simulink model "PUMA_kinematics"  (R2016a)
settings: Solver=VariableStepAuto  StartTime=0.0  StopTime=10.0  RelTol=1e-3
values from neighbouring files (symbols this model uses):
  a2 = 320    [Puma_data.m]
  a3 = 0    [Puma_data.m]
  a4 = 0    [Puma_data.m]
  a5 = 0    [Puma_data.m]
  a6 = 0    [Puma_data.m]
  alpha2 = 0    [Puma_data.m]
  alpha3 = 90    [Puma_data.m]
  alpha4 = -90    [Puma_data.m]
  alpha5 = 90    [Puma_data.m]
  alpha6 = 0    [Puma_data.m]
  ceta2 = 0    [Puma_data.m]
  ceta3 = 0    [Puma_data.m]
  ceta4 = 0    [Puma_data.m]
  ceta5 = 0    [Puma_data.m]
  ceta6 = 0    [Puma_data.m]
  d2 = -55    [Puma_data.m]
  d3 = 0    [Puma_data.m]
  d4 = 350    [Puma_data.m]
  d5 = 0    [Puma_data.m]
  d6 = 140    [Puma_data.m]
undefined symbols (not defined in the file or in its folder): a1, alpha1, ceta1, d1
settings Model: Creator=Amr  LastModifiedBy=Amr

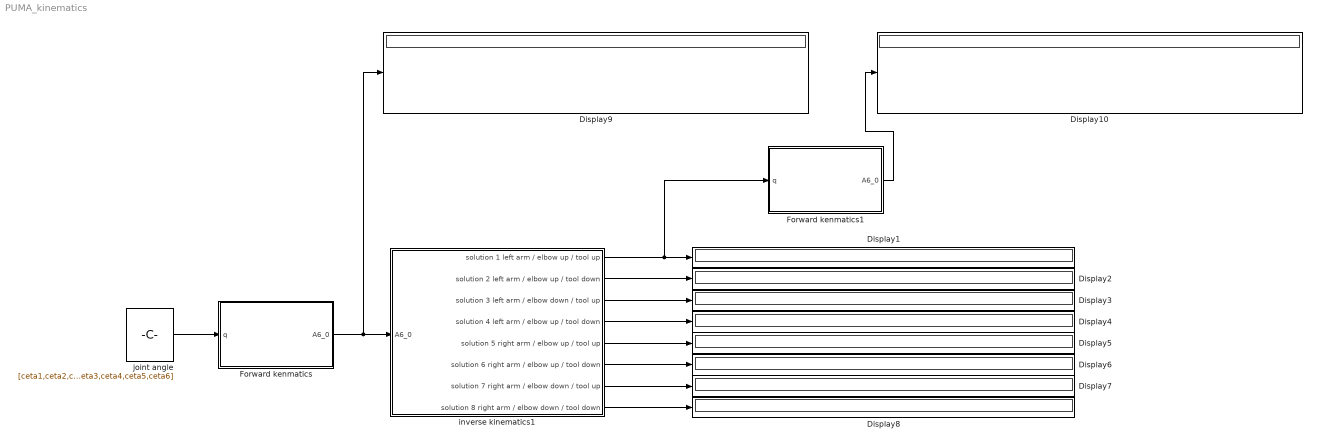
== system PUMA_kinematics ==
  Display{1..10} (10 alike) : Display
  Forward kenmatics : Subsystem
  Forward kenmatics1 : Subsystem
  inverse kinematics1 : Subsystem
  joint angle : Constant  Value=[ceta1,ceta2,ceta3,ceta4,ceta5,ceta6]
  wires:
  joint angle/1 -> Forward kenmatics/1(q)
  inverse kinematics1/1(solution 1 left arm / elbow up / tool up) -> Forward kenmatics1/1(q), Display1/1
  inverse kinematics1/4(solution 4 left arm / elbow up / tool down) -> Display4/1
  inverse kinematics1/3(solution 3 left arm / elbow down / tool up) -> Display3/1
  inverse kinematics1/2(solution 2 left arm / elbow up / tool down) -> Display2/1
  inverse kinematics1/6(solution 6 right arm / elbow up / tool down) -> Display6/1
  inverse kinematics1/7(solution 7 right arm / elbow down / tool up) -> Display7/1
  Forward kenmatics/1(A6_0) -> Display9/1, inverse kinematics1/1(A6_0)
  inverse kinematics1/8(solution 8 right arm / elbow down / tool down) -> Display8/1
  Forward kenmatics1/1(A6_0) -> Display10/1
  inverse kinematics1/5(solution 5 right arm / elbow up / tool up) -> Display5/1

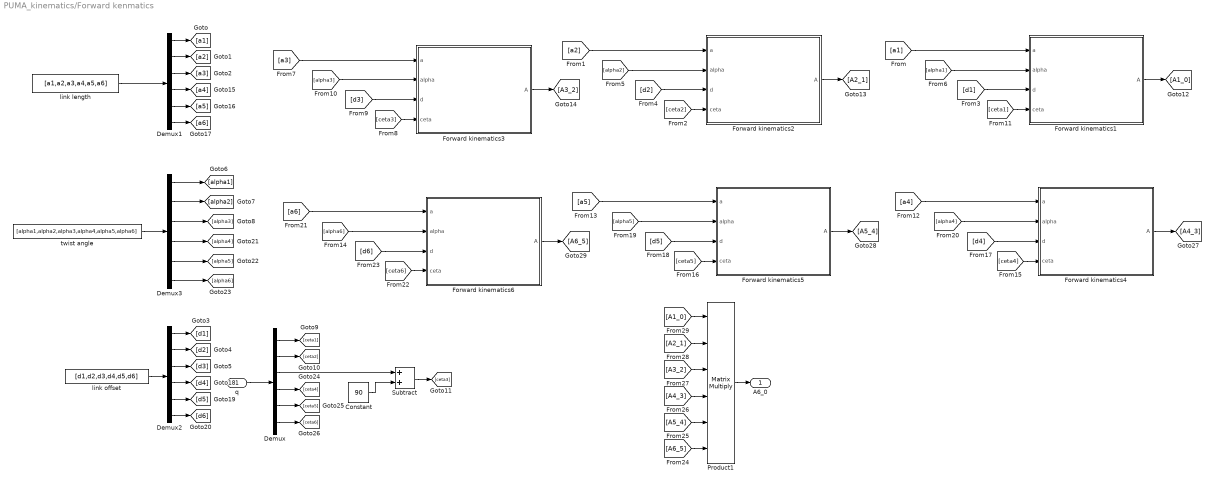
== system PUMA_kinematics/Forward kenmatics ==
  q : Inport
  " Forward kinematics1" : MATLAB Function  TreatAsAtomicUnit=on
  " Forward kinematics2" : MATLAB Function  TreatAsAtomicUnit=on
  " Forward kinematics3" : MATLAB Function  TreatAsAtomicUnit=on
  " Forward kinematics4" : MATLAB Function  TreatAsAtomicUnit=on
  " Forward kinematics5" : MATLAB Function  TreatAsAtomicUnit=on
  " Forward kinematics6" : MATLAB Function  TreatAsAtomicUnit=on
  Constant : Constant  Value=90
  Demux{,1..3} (4 alike) : Demux  Outputs=6
  Product1 : Product  Inputs=6  Multiplication=Matrix(*)
  Subtract : Sum
  link length : Constant  Value=[a1,a2,a3,a4,a5,a6]
  link offset : Constant  Value=[d1,d2,d3,d4,d5,d6]
  twist angle : Constant  Value=[alpha1,alpha2,alpha3,alpha4,alpha5,alpha6]
  A6_0 : Outport
  wires:
  Demux2/4 -> [d4]
  " Forward kinematics3"/1(A) -> [A3_2]
  Demux2/6 -> [d6]
  Demux1/6 -> [a6]
  Demux1/4 -> [a4]
  Demux/4 -> [ceta4]
  Demux/5 -> [ceta5]
  Demux1/5 -> [a5]
  " Forward kinematics1"/1(A) -> [A1_0]
  [d2] -> " Forward kinematics2"/3(d)
  [a2] -> " Forward kinematics2"/1(a)
  [alpha2] -> " Forward kinematics2"/2(alpha)
  [ceta2] -> " Forward kinematics2"/4(ceta)
  [ceta4] -> " Forward kinematics4"/4(ceta)
  [a5] -> " Forward kinematics5"/1(a)
  [a6] -> " Forward kinematics6"/1(a)
  [d6] -> " Forward kinematics6"/3(d)
  [alpha4] -> " Forward kinematics4"/2(alpha)
  [a4] -> " Forward kinematics4"/1(a)
  [alpha5] -> " Forward kinematics5"/2(alpha)
  [ceta5] -> " Forward kinematics5"/4(ceta)
  [d4] -> " Forward kinematics4"/3(d)
  [d5] -> " Forward kinematics5"/3(d)
  [alpha6] -> " Forward kinematics6"/2(alpha)
  " Forward kinematics6"/1(A) -> [A6_5]
  " Forward kinematics5"/1(A) -> [A5_4]
  " Forward kinematics4"/1(A) -> [A4_3]
  [ceta6] -> " Forward kinematics6"/4(ceta)
  Demux3/6 -> [alpha6]
  Demux2/5 -> [d5]
  " Forward kinematics2"/1(A) -> [A2_1]
  Demux3/5 -> [alpha5]
  Demux3/4 -> [alpha4]
  Demux/6 -> [ceta6]
  [d3] -> " Forward kinematics3"/3(d)
  [ceta3] -> " Forward kinematics3"/4(ceta)
  [a3] -> " Forward kinematics3"/1(a)
  [alpha3] -> " Forward kinematics3"/2(alpha)
  Demux1/1 -> [a1]
  Demux1/2 -> [a2]
  q/1 -> Demux/1
  Demux1/3 -> [a3]
  link offset/1 -> Demux2/1
  Demux2/1 -> [d1]
  Product1/1 -> A6_0/1
  Demux/1 -> [ceta1]
  [ceta1] -> " Forward kinematics1"/4(ceta)
  twist angle/1 -> Demux3/1
  Demux3/1 -> [alpha1]
  Demux2/3 -> [d3]
  [a1] -> " Forward kinematics1"/1(a)
  Demux/2 -> [ceta2]
  Demux2/2 -> [d2]
  [d1] -> " Forward kinematics1"/3(d)
  link length/1 -> Demux1/1
  Demux3/2 -> [alpha2]
  [alpha1] -> " Forward kinematics1"/2(alpha)
  Demux3/3 -> [alpha3]
  [A5_4] -> Product1/5
  [A6_5] -> Product1/6
  [A1_0] -> Product1/1
  [A2_1] -> Product1/2
  [A4_3] -> Product1/4
  Constant/1 -> Subtract/2
  Subtract/1 -> [ceta3]
  Demux/3 -> Subtract/1
  [A3_2] -> Product1/3

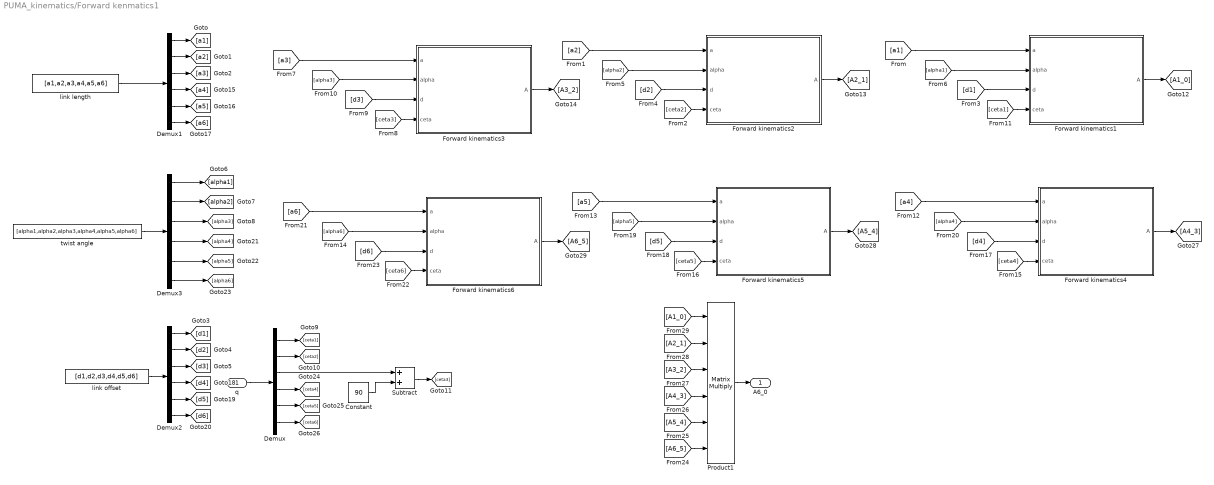
== system PUMA_kinematics/Forward kenmatics1 ==
  q : Inport
  " Forward kinematics1" : MATLAB Function  TreatAsAtomicUnit=on
  " Forward kinematics2" : MATLAB Function  TreatAsAtomicUnit=on
  " Forward kinematics3" : MATLAB Function  TreatAsAtomicUnit=on
  " Forward kinematics4" : MATLAB Function  TreatAsAtomicUnit=on
  " Forward kinematics5" : MATLAB Function  TreatAsAtomicUnit=on
  " Forward kinematics6" : MATLAB Function  TreatAsAtomicUnit=on
  Constant : Constant  Value=90
  Demux{,1..3} (4 alike) : Demux  Outputs=6
  Product1 : Product  Inputs=6  Multiplication=Matrix(*)
  Subtract : Sum
  link length : Constant  Value=[a1,a2,a3,a4,a5,a6]
  link offset : Constant  Value=[d1,d2,d3,d4,d5,d6]
  twist angle : Constant  Value=[alpha1,alpha2,alpha3,alpha4,alpha5,alpha6]
  A6_0 : Outport
  wires:
  Demux2/4 -> [d4]
  " Forward kinematics3"/1(A) -> [A3_2]
  Demux2/6 -> [d6]
  Demux1/6 -> [a6]
  Demux1/4 -> [a4]
  Demux/4 -> [ceta4]
  Demux/5 -> [ceta5]
  Demux1/5 -> [a5]
  " Forward kinematics1"/1(A) -> [A1_0]
  [d2] -> " Forward kinematics2"/3(d)
  [a2] -> " Forward kinematics2"/1(a)
  [alpha2] -> " Forward kinematics2"/2(alpha)
  [ceta2] -> " Forward kinematics2"/4(ceta)
  [ceta4] -> " Forward kinematics4"/4(ceta)
  [a5] -> " Forward kinematics5"/1(a)
  [a6] -> " Forward kinematics6"/1(a)
  [d6] -> " Forward kinematics6"/3(d)
  [alpha4] -> " Forward kinematics4"/2(alpha)
  [a4] -> " Forward kinematics4"/1(a)
  [alpha5] -> " Forward kinematics5"/2(alpha)
  [ceta5] -> " Forward kinematics5"/4(ceta)
  [d4] -> " Forward kinematics4"/3(d)
  [d5] -> " Forward kinematics5"/3(d)
  [alpha6] -> " Forward kinematics6"/2(alpha)
  " Forward kinematics6"/1(A) -> [A6_5]
  " Forward kinematics5"/1(A) -> [A5_4]
  " Forward kinematics4"/1(A) -> [A4_3]
  [ceta6] -> " Forward kinematics6"/4(ceta)
  Demux3/6 -> [alpha6]
  Demux2/5 -> [d5]
  " Forward kinematics2"/1(A) -> [A2_1]
  Demux3/5 -> [alpha5]
  Demux3/4 -> [alpha4]
  Demux/6 -> [ceta6]
  [d3] -> " Forward kinematics3"/3(d)
  [ceta3] -> " Forward kinematics3"/4(ceta)
  [a3] -> " Forward kinematics3"/1(a)
  [alpha3] -> " Forward kinematics3"/2(alpha)
  Demux1/1 -> [a1]
  Demux1/2 -> [a2]
  q/1 -> Demux/1
  Demux1/3 -> [a3]
  link offset/1 -> Demux2/1
  Demux2/1 -> [d1]
  Product1/1 -> A6_0/1
  Demux/1 -> [ceta1]
  [ceta1] -> " Forward kinematics1"/4(ceta)
  twist angle/1 -> Demux3/1
  Demux3/1 -> [alpha1]
  Demux2/3 -> [d3]
  [a1] -> " Forward kinematics1"/1(a)
  Demux/2 -> [ceta2]
  Demux2/2 -> [d2]
  [d1] -> " Forward kinematics1"/3(d)
  link length/1 -> Demux1/1
  Demux3/2 -> [alpha2]
  [alpha1] -> " Forward kinematics1"/2(alpha)
  Demux3/3 -> [alpha3]
  [A5_4] -> Product1/5
  [A6_5] -> Product1/6
  [A1_0] -> Product1/1
  [A2_1] -> Product1/2
  [A4_3] -> Product1/4
  Constant/1 -> Subtract/2
  Subtract/1 -> [ceta3]
  Demux/3 -> Subtract/1
  [A3_2] -> Product1/3

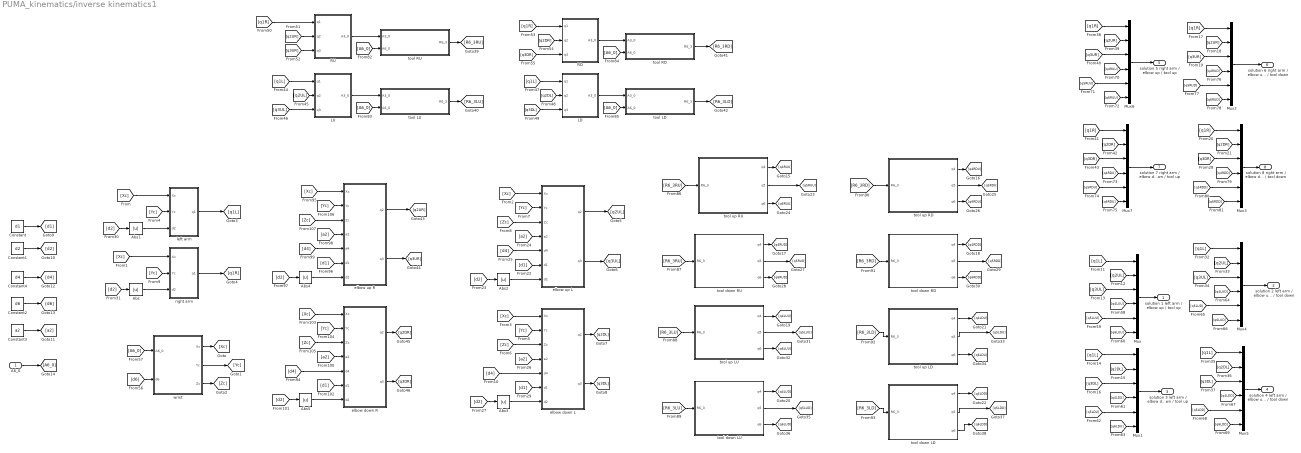
== system PUMA_kinematics/inverse kinematics1 ==
  A6_0 : Inport
  Abs{,1..5} (6 alike) : Abs
  Constant : Constant  Value=d1
  Constant1 : Constant  Value=d2
  Constant2 : Constant  Value=d6
  Constant3 : Constant  Value=a2
  Constant4 : Constant  Value=d4
  LD : Subsystem
  LU : Subsystem
  Mux{,1..7} (8 alike) : Mux  Inputs=6
  RD : Subsystem
  RU : Subsystem
  elbow down L : MATLAB Function  TreatAsAtomicUnit=on
  elbow down R : MATLAB Function  TreatAsAtomicUnit=on
  elbow up L : MATLAB Function  TreatAsAtomicUnit=on
  elbow up R : MATLAB Function  TreatAsAtomicUnit=on
  left arm : MATLAB Function  TreatAsAtomicUnit=on
  right arm : MATLAB Function  TreatAsAtomicUnit=on
  tool LD : MATLAB Function  TreatAsAtomicUnit=on
  tool LU : MATLAB Function  TreatAsAtomicUnit=on
  tool RD : MATLAB Function  TreatAsAtomicUnit=on
  tool RU : MATLAB Function  TreatAsAtomicUnit=on
  tool down LD : MATLAB Function  TreatAsAtomicUnit=on
  tool down LU : MATLAB Function  TreatAsAtomicUnit=on
  tool down RD : MATLAB Function  TreatAsAtomicUnit=on
  tool down RU : MATLAB Function  TreatAsAtomicUnit=on
  tool up LD : MATLAB Function  TreatAsAtomicUnit=on
  tool up LU : MATLAB Function  TreatAsAtomicUnit=on
  tool up RD : MATLAB Function  TreatAsAtomicUnit=on
  tool up RU : MATLAB Function  TreatAsAtomicUnit=on
  wrist : MATLAB Function  TreatAsAtomicUnit=on
  solution 1 left arm / elbow up / tool up : Outport
  solution 2 left arm / elbow up / tool down : Outport  Port=2
  solution 3 left arm / elbow down / tool up : Outport  Port=3
  solution 4 left arm / elbow up / tool down : Outport  Port=4
  solution 5 right arm / elbow up / tool up : Outport  Port=5
  solution 6 right arm / elbow up / tool down : Outport  Port=6
  solution 7 right arm / elbow down / tool up : Outport  Port=7
  solution 8 right arm / elbow down / tool down : Outport  Port=8
  wires:
  [Yc] -> right arm/2(Yc)
  left arm/1(q1) -> [q1L]
  [Yc] -> left arm/2(Yc)
  [d6] -> wrist/2(d6)
  wrist/2(Yc) -> [Yc]
  Constant/1 -> [d1]
  Constant3/1 -> [a2]
  [A6_0] -> wrist/1(A6_0)
  A6_0/1 -> [A6_0]
  Constant4/1 -> [d4]
  Constant1/1 -> [d2]
  Constant2/1 -> [d6]
  right arm/1(q1) -> [q1R]
  wrist/3(Zc) -> [Zc]
  [Xc] -> right arm/1(Xc)
  [Xc] -> left arm/1(Xc)
  wrist/1(Xc) -> [Xc]
  [d2] -> Abs/1
  Abs/1 -> right arm/3(d2)
  [d2] -> Abs1/1
  Abs1/1 -> left arm/3(d2)
  [d4] -> elbow up L/5(d4)
  [Xc] -> elbow up L/1(Xc)
  [d1] -> elbow up L/6(d1)
  [a2] -> elbow up L/4(a2)
  [Zc] -> elbow up L/3(Zc)
  [Yc] -> elbow up L/2(Yc)
  [d2] -> Abs2/1
  Abs2/1 -> elbow up L/7(d2)
  elbow up L/2(q3) -> [q3UL]
  elbow up L/1(q2) -> [q2UL]
  elbow down L/2(q3) -> [q3DL]
  elbow down L/1(q2) -> [q2DL]
  [a2] -> elbow down L/4(a2)
  [d4] -> elbow down L/5(d4)
  [Xc] -> elbow down L/1(Xc)
  [Yc] -> elbow down L/2(Yc)
  [d1] -> elbow down L/6(d1)
  [Zc] -> elbow down L/3(Zc)
  Abs3/1 -> elbow down L/7(d2)
  [d2] -> Abs3/1
  [q3UL] -> LU/3(q3)
  [q1R] -> RD/1(q1)
  [q3DR] -> RD/3(q3)
  [q2DR] -> RD/2(q2)
  [q2UL] -> LU/2(q2)
  RU/1(A3_0) -> tool RU/1(A3_0)
  LU/1(A3_0) -> tool LU/1(A3_0)
  RD/1(A3_0) -> tool RD/1(A3_0)
  LD/1(A3_0) -> tool LD/1(A3_0)
  [A6_0] -> tool RU/2(A6_0)
  [A6_0] -> tool LU/2(A6_0)
  [A6_0] -> tool RD/2(A6_0)
  [A6_0] -> tool LD/2(A6_0)
  tool RU/1(R6_3) -> [R6_3RU]
  tool LU/1(R6_3) -> [R6_3LU]
  [q1L] -> LU/1(q1)
  [q1R] -> RU/1(q1)
  [q2UR] -> RU/2(q2)
  [q3UR] -> RU/3(q3)
  [q3DL] -> LD/3(q3)
  [q1L] -> LD/1(q1)
  [q2DL] -> LD/2(q2)
  tool RD/1(R6_3) -> [R6_3RD]
  tool up RU/1(q4) -> [q4RUU]
  tool up RU/2(q5) -> [q5RUU]
  tool up RU/3(q6) -> [q6RUU]
  tool LD/1(R6_3) -> [R6_3LD]
  [R6_3RU] -> tool up RU/1(R6_3)
  tool up LD/2(q5) -> [q5LDU]
  tool up LD/1(q4) -> [q4LDU]
  tool down LD/2(q5) -> [q5LDD]
  tool up LD/3(q6) -> [q6LDU]
  tool down RD/1(q4) -> [q4RDD]
  tool down RD/2(q5) -> [q5RDD]
  tool down RD/3(q6) -> [q6RDD]
  tool up RD/1(q4) -> [q4RDU]
  tool up RD/3(q6) -> [q6RDU]
  tool up RD/2(q5) -> [q5RDU]
  [R6_3RD] -> tool down RD/1(R6_3)
  [R6_3RD] -> tool up RD/1(R6_3)
  [R6_3LD] -> tool up LD/1(R6_3)
  [R6_3LD] -> tool down LD/1(R6_3)
  tool down LU/1(q4) -> [q4LUD]
  tool down LU/2(q5) -> [q5LUD]
  tool down LU/3(q6) -> [q6LUD]
  tool down RU/1(q4) -> [q4RUD]
  tool up LU/1(q4) -> [q4LUU]
  tool down RU/3(q6) -> [q6RUD]
  tool down RU/2(q5) -> [q5RUD]
  tool up LU/2(q5) -> [q5LUU]
  tool up LU/3(q6) -> [q6LUU]
  [R6_3RU] -> tool down RU/1(R6_3)
  [R6_3LU] -> tool up LU/1(R6_3)
  [R6_3LU] -> tool down LU/1(R6_3)
  [q3DL] -> Mux1/3
  [q3UR] -> Mux2/3
  [q2UR] -> Mux2/2
  [q1R] -> Mux2/1
  [q4LDD] -> Mux5/4
  [q5LDD] -> Mux5/5
  [q6LDD] -> Mux5/6
  [q4LUD] -> Mux4/4
  [q5LUU] -> Mux/5
  [q4LUU] -> Mux/4
  [q6LUU] -> Mux/6
  [q5LUD] -> Mux4/5
  [q5RUU] -> Mux6/5
  [q6LUD] -> Mux4/6
  [q4RUU] -> Mux6/4
  [q6RUU] -> Mux6/6
  [q4RUD] -> Mux2/4
  [q6RUD] -> Mux2/6
  [q5RUD] -> Mux2/5
  [q1R] -> Mux3/1
  [q2DL] -> Mux1/2
  [q3UL] -> Mux/3
  [q5LDU] -> Mux1/5
  [q6LDU] -> Mux1/6
  [q4LDU] -> Mux1/4
  [q3DR] -> Mux3/3
  Mux/1 -> solution 1 left arm / elbow up / tool up/1
  [q1L] -> Mux1/1
  [q3DR] -> Mux7/3
  [q2DL] -> Mux5/2
  [q1R] -> Mux7/1
  [q3UR] -> Mux6/3
  [q1R] -> Mux6/1
  [q1L] -> Mux5/1
  [q2DR] -> Mux7/2
  [q3UL] -> Mux4/3
  [q2UR] -> Mux6/2
  [q3DL] -> Mux5/3
  [q1L] -> Mux4/1
  [q2UL] -> Mux4/2
  [q2DR] -> Mux3/2
  [q1L] -> Mux/1
  [q2UL] -> Mux/2
  Mux4/1 -> solution 2 left arm / elbow up / tool down/1
  Mux1/1 -> solution 3 left arm / elbow down / tool up/1
  Mux5/1 -> solution 4 left arm / elbow up / tool down/1
  Mux6/1 -> solution 5 right arm / elbow up / tool up/1
  Mux2/1 -> solution 6 right arm / elbow up / tool down/1
  Mux7/1 -> solution 7 right arm / elbow down / tool up/1
  Mux3/1 -> solution 8 right arm / elbow down / tool down/1
  [q4RDU] -> Mux7/4
  [q5RDU] -> Mux7/5
  [q6RDU] -> Mux7/6
  [q6RDD] -> Mux3/6
  [q5RDD] -> Mux3/5
  [q4RDD] -> Mux3/4
  tool down LD/1(q4) -> [q4LDD]
  tool down LD/3(q6) -> [q6LDD]
  [d4] -> elbow up R/5(d4)
  [Xc] -> elbow up R/1(Xc)
  [d1] -> elbow up R/6(d1)
  [a2] -> elbow up R/4(a2)
  [Zc] -> elbow up R/3(Zc)
  [Yc] -> elbow up R/2(Yc)
  [d2] -> Abs4/1
  Abs4/1 -> elbow up R/7(d2)
  elbow up R/2(q3) -> [q3UR]
  elbow up R/1(q2) -> [q2UR]
  elbow down R/2(q3) -> [q3DR]
  elbow down R/1(q2) -> [q2DR]
  [a2] -> elbow down R/4(a2)
  [d4] -> elbow down R/5(d4)
  [Xc] -> elbow down R/1(Xc)
  [Yc] -> elbow down R/2(Yc)
  [d1] -> elbow down R/6(d1)
  [Zc] -> elbow down R/3(Zc)
  Abs5/1 -> elbow down R/7(d2)
  [d2] -> Abs5/1

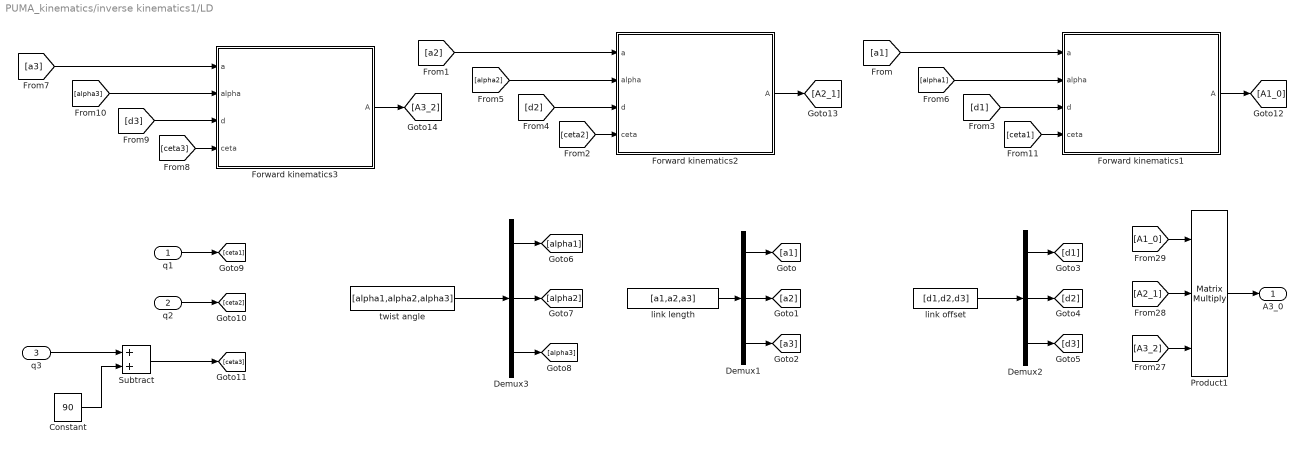
== system PUMA_kinematics/inverse kinematics1/LD ==
  q1 : Inport
  q2 : Inport  Port=2
  q3 : Inport  Port=3
  " Forward kinematics1" : MATLAB Function  TreatAsAtomicUnit=on
  " Forward kinematics2" : MATLAB Function  TreatAsAtomicUnit=on
  " Forward kinematics3" : MATLAB Function  TreatAsAtomicUnit=on
  Constant : Constant  Value=90
  Demux1 : Demux  Outputs=3
  Demux2 : Demux  Outputs=3
  Demux3 : Demux  Outputs=3
  Product1 : Product  Inputs=3  Multiplication=Matrix(*)
  Subtract : Sum
  link length : Constant  Value=[a1,a2,a3]
  link offset : Constant  Value=[d1,d2,d3]
  twist angle : Constant  Value=[alpha1,alpha2,alpha3]
  A3_0 : Outport
  wires:
  " Forward kinematics3"/1(A) -> [A3_2]
  " Forward kinematics1"/1(A) -> [A1_0]
  [d2] -> " Forward kinematics2"/3(d)
  [a2] -> " Forward kinematics2"/1(a)
  [alpha2] -> " Forward kinematics2"/2(alpha)
  [ceta2] -> " Forward kinematics2"/4(ceta)
  " Forward kinematics2"/1(A) -> [A2_1]
  [d3] -> " Forward kinematics3"/3(d)
  [ceta3] -> " Forward kinematics3"/4(ceta)
  [a3] -> " Forward kinematics3"/1(a)
  [alpha3] -> " Forward kinematics3"/2(alpha)
  Demux1/1 -> [a1]
  Demux1/2 -> [a2]
  Demux1/3 -> [a3]
  link offset/1 -> Demux2/1
  Demux2/1 -> [d1]
  Product1/1 -> A3_0/1
  [ceta1] -> " Forward kinematics1"/4(ceta)
  twist angle/1 -> Demux3/1
  Demux3/1 -> [alpha1]
  Demux2/3 -> [d3]
  [a1] -> " Forward kinematics1"/1(a)
  Demux2/2 -> [d2]
  [d1] -> " Forward kinematics1"/3(d)
  link length/1 -> Demux1/1
  Demux3/2 -> [alpha2]
  [alpha1] -> " Forward kinematics1"/2(alpha)
  Demux3/3 -> [alpha3]
  [A3_2] -> Product1/3
  [A1_0] -> Product1/1
  [A2_1] -> Product1/2
  q1/1 -> [ceta1]
  q2/1 -> [ceta2]
  Constant/1 -> Subtract/2
  Subtract/1 -> [ceta3]
  q3/1 -> Subtract/1

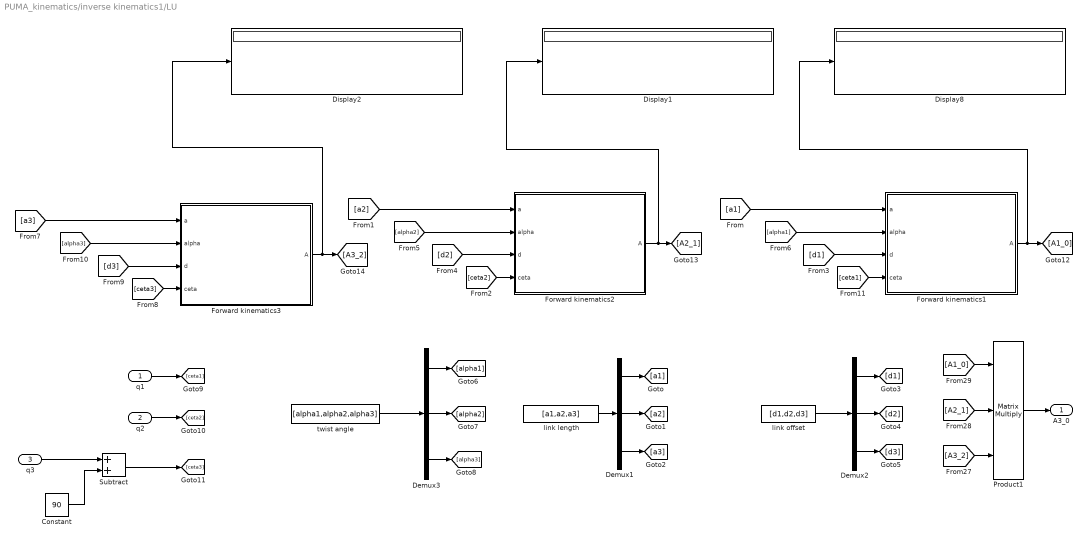
== system PUMA_kinematics/inverse kinematics1/LU ==
  q1 : Inport
  q2 : Inport  Port=2
  q3 : Inport  Port=3
  " Forward kinematics1" : MATLAB Function  TreatAsAtomicUnit=on
  " Forward kinematics2" : MATLAB Function  TreatAsAtomicUnit=on
  " Forward kinematics3" : MATLAB Function  TreatAsAtomicUnit=on
  Constant : Constant  Value=90
  Demux1 : Demux  Outputs=3
  Demux2 : Demux  Outputs=3
  Demux3 : Demux  Outputs=3
  Display1 : Display
  Display2 : Display
  Display8 : Display
  Product1 : Product  Inputs=3  Multiplication=Matrix(*)
  Subtract : Sum
  link length : Constant  Value=[a1,a2,a3]
  link offset : Constant  Value=[d1,d2,d3]
  twist angle : Constant  Value=[alpha1,alpha2,alpha3]
  A3_0 : Outport
  wires:
  " Forward kinematics3"/1(A) -> Display2/1, [A3_2]
  " Forward kinematics1"/1(A) -> Display8/1, [A1_0]
  [d2] -> " Forward kinematics2"/3(d)
  [a2] -> " Forward kinematics2"/1(a)
  [alpha2] -> " Forward kinematics2"/2(alpha)
  [ceta2] -> " Forward kinematics2"/4(ceta)
  [d3] -> " Forward kinematics3"/3(d)
  [ceta3] -> " Forward kinematics3"/4(ceta)
  [a3] -> " Forward kinematics3"/1(a)
  [alpha3] -> " Forward kinematics3"/2(alpha)
  Demux1/1 -> [a1]
  Demux1/2 -> [a2]
  Demux1/3 -> [a3]
  link offset/1 -> Demux2/1
  Demux2/1 -> [d1]
  Product1/1 -> A3_0/1
  [ceta1] -> " Forward kinematics1"/4(ceta)
  twist angle/1 -> Demux3/1
  Demux3/1 -> [alpha1]
  Demux2/3 -> [d3]
  [a1] -> " Forward kinematics1"/1(a)
  Demux2/2 -> [d2]
  [d1] -> " Forward kinematics1"/3(d)
  link length/1 -> Demux1/1
  Demux3/2 -> [alpha2]
  [alpha1] -> " Forward kinematics1"/2(alpha)
  Demux3/3 -> [alpha3]
  [A3_2] -> Product1/3
  [A1_0] -> Product1/1
  [A2_1] -> Product1/2
  q1/1 -> [ceta1]
  q2/1 -> [ceta2]
  Constant/1 -> Subtract/2
  Subtract/1 -> [ceta3]
  q3/1 -> Subtract/1
  " Forward kinematics2"/1(A) -> [A2_1], Display1/1

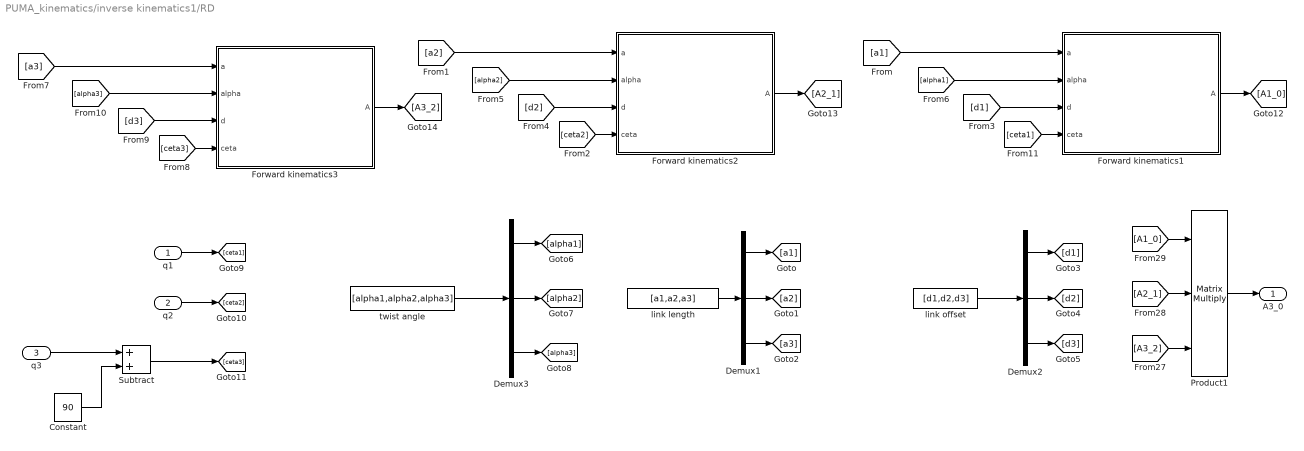
== system PUMA_kinematics/inverse kinematics1/RD ==
  q1 : Inport
  q2 : Inport  Port=2
  q3 : Inport  Port=3
  " Forward kinematics1" : MATLAB Function  TreatAsAtomicUnit=on
  " Forward kinematics2" : MATLAB Function  TreatAsAtomicUnit=on
  " Forward kinematics3" : MATLAB Function  TreatAsAtomicUnit=on
  Constant : Constant  Value=90
  Demux1 : Demux  Outputs=3
  Demux2 : Demux  Outputs=3
  Demux3 : Demux  Outputs=3
  Product1 : Product  Inputs=3  Multiplication=Matrix(*)
  Subtract : Sum
  link length : Constant  Value=[a1,a2,a3]
  link offset : Constant  Value=[d1,d2,d3]
  twist angle : Constant  Value=[alpha1,alpha2,alpha3]
  A3_0 : Outport
  wires:
  " Forward kinematics3"/1(A) -> [A3_2]
  " Forward kinematics1"/1(A) -> [A1_0]
  [d2] -> " Forward kinematics2"/3(d)
  [a2] -> " Forward kinematics2"/1(a)
  [alpha2] -> " Forward kinematics2"/2(alpha)
  [ceta2] -> " Forward kinematics2"/4(ceta)
  " Forward kinematics2"/1(A) -> [A2_1]
  [d3] -> " Forward kinematics3"/3(d)
  [ceta3] -> " Forward kinematics3"/4(ceta)
  [a3] -> " Forward kinematics3"/1(a)
  [alpha3] -> " Forward kinematics3"/2(alpha)
  Demux1/1 -> [a1]
  Demux1/2 -> [a2]
  Demux1/3 -> [a3]
  link offset/1 -> Demux2/1
  Demux2/1 -> [d1]
  Product1/1 -> A3_0/1
  [ceta1] -> " Forward kinematics1"/4(ceta)
  twist angle/1 -> Demux3/1
  Demux3/1 -> [alpha1]
  Demux2/3 -> [d3]
  [a1] -> " Forward kinematics1"/1(a)
  Demux2/2 -> [d2]
  [d1] -> " Forward kinematics1"/3(d)
  link length/1 -> Demux1/1
  Demux3/2 -> [alpha2]
  [alpha1] -> " Forward kinematics1"/2(alpha)
  Demux3/3 -> [alpha3]
  [A3_2] -> Product1/3
  [A1_0] -> Product1/1
  [A2_1] -> Product1/2
  q1/1 -> [ceta1]
  q2/1 -> [ceta2]
  Constant/1 -> Subtract/2
  Subtract/1 -> [ceta3]
  q3/1 -> Subtract/1

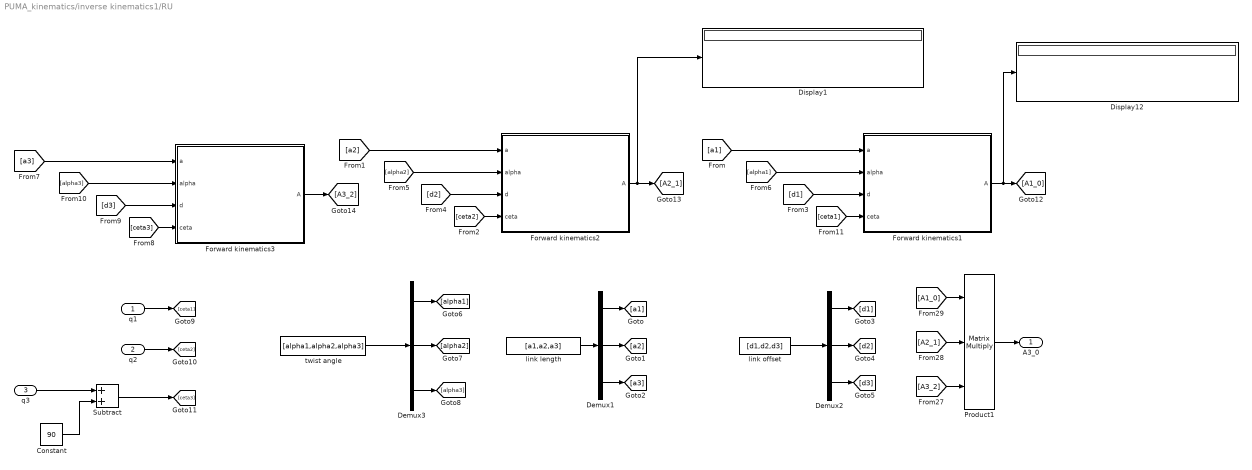
== system PUMA_kinematics/inverse kinematics1/RU ==
  q1 : Inport
  q2 : Inport  Port=2
  q3 : Inport  Port=3
  " Forward kinematics1" : MATLAB Function  TreatAsAtomicUnit=on
  " Forward kinematics2" : MATLAB Function  TreatAsAtomicUnit=on
  " Forward kinematics3" : MATLAB Function  TreatAsAtomicUnit=on
  Constant : Constant  Value=90
  Demux1 : Demux  Outputs=3
  Demux2 : Demux  Outputs=3
  Demux3 : Demux  Outputs=3
  Display1 : Display
  Display12 : Display
  Product1 : Product  Inputs=3  Multiplication=Matrix(*)
  Subtract : Sum
  link length : Constant  Value=[a1,a2,a3]
  link offset : Constant  Value=[d1,d2,d3]
  twist angle : Constant  Value=[alpha1,alpha2,alpha3]
  A3_0 : Outport
  wires:
  " Forward kinematics3"/1(A) -> [A3_2]
  " Forward kinematics1"/1(A) -> Display12/1, [A1_0]
  [d2] -> " Forward kinematics2"/3(d)
  [a2] -> " Forward kinematics2"/1(a)
  [alpha2] -> " Forward kinematics2"/2(alpha)
  [ceta2] -> " Forward kinematics2"/4(ceta)
  " Forward kinematics2"/1(A) -> Display1/1, [A2_1]
  [d3] -> " Forward kinematics3"/3(d)
  [ceta3] -> " Forward kinematics3"/4(ceta)
  [a3] -> " Forward kinematics3"/1(a)
  [alpha3] -> " Forward kinematics3"/2(alpha)
  Demux1/1 -> [a1]
  Demux1/2 -> [a2]
  Demux1/3 -> [a3]
  link offset/1 -> Demux2/1
  Demux2/1 -> [d1]
  Product1/1 -> A3_0/1
  [ceta1] -> " Forward kinematics1"/4(ceta)
  twist angle/1 -> Demux3/1
  Demux3/1 -> [alpha1]
  Demux2/3 -> [d3]
  [a1] -> " Forward kinematics1"/1(a)
  Demux2/2 -> [d2]
  [d1] -> " Forward kinematics1"/3(d)
  link length/1 -> Demux1/1
  Demux3/2 -> [alpha2]
  [alpha1] -> " Forward kinematics1"/2(alpha)
  Demux3/3 -> [alpha3]
  [A3_2] -> Product1/3
  [A1_0] -> Product1/1
  [A2_1] -> Product1/2
  q1/1 -> [ceta1]
  q2/1 -> [ceta2]
  Constant/1 -> Subtract/2
  Subtract/1 -> [ceta3]
  q3/1 -> Subtract/1

== matlab function PUMA_kinematics/Forward kenmatics/ Forward kinematics2 ==
  data: a input; alpha input; A output; d input; ceta input

function  A=fk_transformation_matrix(a,alpha,d,ceta )


A=[cosd(ceta) , (-1*sind(ceta)*cosd(alpha)) , (sind(ceta)*sind(alpha)) , (a*cosd(ceta)) ;...........................
    sind(ceta) , (cosd(ceta)*cosd(alpha)) ,(-1*cosd(ceta)*sind(alpha)) , (a*sind(ceta)) ;............................
    0 , sind(alpha) , cosd(alpha) , d ;..................................................................................
    0,0,0,1];

== matlab function PUMA_kinematics/Forward kenmatics/ Forward kinematics3 ==
  data: a input; alpha input; A output; d input; ceta input

function  A=fk_transformation_matrix(a,alpha,d,ceta )


A=[cosd(ceta) , (-1*sind(ceta)*cosd(alpha)) , (sind(ceta)*sind(alpha)) , (a*cosd(ceta)) ;...........................
    sind(ceta) , (cosd(ceta)*cosd(alpha)) ,(-1*cosd(ceta)*sind(alpha)) , (a*sind(ceta)) ;............................
    0 , sind(alpha) , cosd(alpha) , d ;..................................................................................
    0,0,0,1];

== matlab function PUMA_kinematics/Forward kenmatics/ Forward kinematics4 ==
  data: a input; alpha input; A output; d input; ceta input

function  A=fk_transformation_matrix(a,alpha,d,ceta )


A=[cosd(ceta) , (-1*sind(ceta)*cosd(alpha)) , (sind(ceta)*sind(alpha)) , (a*cosd(ceta)) ;...........................
    sind(ceta) , (cosd(ceta)*cosd(alpha)) ,(-1*cosd(ceta)*sind(alpha)) , (a*sind(ceta)) ;............................
    0 , sind(alpha) , cosd(alpha) , d ;..................................................................................
    0,0,0,1];

== matlab function PUMA_kinematics/Forward kenmatics/ Forward kinematics5 ==
  data: a input; alpha input; A output; d input; ceta input

function  A=fk_transformation_matrix(a,alpha,d,ceta )


A=[cosd(ceta) , (-1*sind(ceta)*cosd(alpha)) , (sind(ceta)*sind(alpha)) , (a*cosd(ceta)) ;...........................
    sind(ceta) , (cosd(ceta)*cosd(alpha)) ,(-1*cosd(ceta)*sind(alpha)) , (a*sind(ceta)) ;............................
    0 , sind(alpha) , cosd(alpha) , d ;..................................................................................
    0,0,0,1];

== matlab function PUMA_kinematics/Forward kenmatics/ Forward kinematics6 ==
  data: a input; alpha input; A output; d input; ceta input

function  A=fk_transformation_matrix(a,alpha,d,ceta )


A=[cosd(ceta) , (-1*sind(ceta)*cosd(alpha)) , (sind(ceta)*sind(alpha)) , (a*cosd(ceta)) ;...........................
    sind(ceta) , (cosd(ceta)*cosd(alpha)) ,(-1*cosd(ceta)*sind(alpha)) , (a*sind(ceta)) ;............................
    0 , sind(alpha) , cosd(alpha) , d ;..................................................................................
    0,0,0,1];

== matlab function PUMA_kinematics/inverse kinematics1/elbow up L ==
  data: q2 output; Xc input; Yc input; Zc input; a2 input; d4 input; d1 input; d2 input; q3 output



function [q2,q3]  = elbow_up(Xc,Yc,Zc,a2,d4,d1,d2)


D  = ((Xc^2)+(Yc^2)-(d2^2)+(Zc-d1)^2-(a2^2)-(d4^2))/(2*a2*d4);

q3 = atan2d(-1*(sqrt(1-(D^2))),D);

q2 = atan2d((Zc-d1),sqrt((Xc^2)+(Yc^2)-(d2^2))) - atan2d(d4*sind(q3),a2+d4*cosd(q3));

end

== matlab function PUMA_kinematics/inverse kinematics1/LD/ Forward kinematics1 ==
  data: a input; alpha input; A output; d input; ceta input

function  A=fk_transformation_matrix(a,alpha,d,ceta )


A=[cosd(ceta) , (-1*sind(ceta)*cosd(alpha)) , (sind(ceta)*sind(alpha)) , (a*cosd(ceta)) ;...........................
    sind(ceta) , (cosd(ceta)*cosd(alpha)) ,(-1*cosd(ceta)*sind(alpha)) , (a*sind(ceta)) ;............................
    0 , sind(alpha) , cosd(alpha) , d ;..................................................................................
    0,0,0,1];

== matlab function PUMA_kinematics/inverse kinematics1/LD/ Forward kinematics2 ==
  data: a input; alpha input; A output; d input; ceta input

function  A=fk_transformation_matrix(a,alpha,d,ceta )


A=[cosd(ceta) , (-1*sind(ceta)*cosd(alpha)) , (sind(ceta)*sind(alpha)) , (a*cosd(ceta)) ;...........................
    sind(ceta) , (cosd(ceta)*cosd(alpha)) ,(-1*cosd(ceta)*sind(alpha)) , (a*sind(ceta)) ;............................
    0 , sind(alpha) , cosd(alpha) , d ;..................................................................................
    0,0,0,1];

== matlab function PUMA_kinematics/inverse kinematics1/LD/ Forward kinematics3 ==
  data: a input; alpha input; A output; d input; ceta input

function  A=fk_transformation_matrix(a,alpha,d,ceta )


A=[cosd(ceta) , (-1*sind(ceta)*cosd(alpha)) , (sind(ceta)*sind(alpha)) , (a*cosd(ceta)) ;...........................
    sind(ceta) , (cosd(ceta)*cosd(alpha)) ,(-1*cosd(ceta)*sind(alpha)) , (a*sind(ceta)) ;............................
    0 , sind(alpha) , cosd(alpha) , d ;..................................................................................
    0,0,0,1];

== matlab function PUMA_kinematics/inverse kinematics1/LU/ Forward kinematics1 ==
  data: a input; alpha input; A output; d input; ceta input

function  A=fk_transformation_matrix(a,alpha,d,ceta )


A=[cosd(ceta) , (-1*sind(ceta)*cosd(alpha)) , (sind(ceta)*sind(alpha)) , (a*cosd(ceta)) ;...........................
    sind(ceta) , (cosd(ceta)*cosd(alpha)) ,(-1*cosd(ceta)*sind(alpha)) , (a*sind(ceta)) ;............................
    0 , sind(alpha) , cosd(alpha) , d ;..................................................................................
    0,0,0,1];

== matlab function PUMA_kinematics/inverse kinematics1/LU/ Forward kinematics2 ==
  data: a input; alpha input; A output; d input; ceta input

function  A=fk_transformation_matrix(a,alpha,d,ceta )


A=[cosd(ceta) , (-1*sind(ceta)*cosd(alpha)) , (sind(ceta)*sind(alpha)) , (a*cosd(ceta)) ;...........................
    sind(ceta) , (cosd(ceta)*cosd(alpha)) ,(-1*cosd(ceta)*sind(alpha)) , (a*sind(ceta)) ;............................
    0 , sind(alpha) , cosd(alpha) , d ;..................................................................................
    0,0,0,1];

== matlab function PUMA_kinematics/inverse kinematics1/LU/ Forward kinematics3 ==
  data: a input; alpha input; A output; d input; ceta input

function  A=fk_transformation_matrix(a,alpha,d,ceta )


A=[cosd(ceta) , (-1*sind(ceta)*cosd(alpha)) , (sind(ceta)*sind(alpha)) , (a*cosd(ceta)) ;...........................
    sind(ceta) , (cosd(ceta)*cosd(alpha)) ,(-1*cosd(ceta)*sind(alpha)) , (a*sind(ceta)) ;............................
    0 , sind(alpha) , cosd(alpha) , d ;..................................................................................
    0,0,0,1];

== matlab function PUMA_kinematics/inverse kinematics1/elbow down L ==
  data: Xc input; q2 output; Yc input; Zc input; a2 input; d4 input; d1 input; d2 input; q3 output



function [q2,q3]= elbow_down(Xc,Yc,Zc,a2,d4,d1,d2)


D  = ((Xc^2)+(Yc^2)-(d2^2)+(Zc-d1)^2-(a2^2)-(d4^2))/(2*a2*d4);

q3 = atan2d(sqrt(1-(D^2)),D);

q2 = atan2d((Zc-d1),sqrt((Xc^2)+(Yc^2)-(d2^2))) - atan2d(d4*sind(q3),a2+d4*cosd(q3));

end

== matlab function PUMA_kinematics/Forward kenmatics/ Forward kinematics1 ==
  data: a input; alpha input; A output; d input; ceta input

function  A=fk_transformation_matrix(a,alpha,d,ceta )


A=[cosd(ceta) , (-1*sind(ceta)*cosd(alpha)) , (sind(ceta)*sind(alpha)) , (a*cosd(ceta)) ;...........................
    sind(ceta) , (cosd(ceta)*cosd(alpha)) ,(-1*cosd(ceta)*sind(alpha)) , (a*sind(ceta)) ;............................
    0 , sind(alpha) , cosd(alpha) , d ;..................................................................................
    0,0,0,1];

== matlab function PUMA_kinematics/inverse kinematics1/RD/ Forward kinematics1 ==
  data: a input; alpha input; A output; d input; ceta input

function  A=fk_transformation_matrix(a,alpha,d,ceta )


A=[cosd(ceta) , (-1*sind(ceta)*cosd(alpha)) , (sind(ceta)*sind(alpha)) , (a*cosd(ceta)) ;...........................
    sind(ceta) , (cosd(ceta)*cosd(alpha)) ,(-1*cosd(ceta)*sind(alpha)) , (a*sind(ceta)) ;............................
    0 , sind(alpha) , cosd(alpha) , d ;..................................................................................
    0,0,0,1];

== matlab function PUMA_kinematics/inverse kinematics1/RD/ Forward kinematics2 ==
  data: a input; alpha input; A output; d input; ceta input

function  A=fk_transformation_matrix(a,alpha,d,ceta )


A=[cosd(ceta) , (-1*sind(ceta)*cosd(alpha)) , (sind(ceta)*sind(alpha)) , (a*cosd(ceta)) ;...........................
    sind(ceta) , (cosd(ceta)*cosd(alpha)) ,(-1*cosd(ceta)*sind(alpha)) , (a*sind(ceta)) ;............................
    0 , sind(alpha) , cosd(alpha) , d ;..................................................................................
    0,0,0,1];

== matlab function PUMA_kinematics/inverse kinematics1/RD/ Forward kinematics3 ==
  data: a input; alpha input; A output; d input; ceta input

function  A=fk_transformation_matrix(a,alpha,d,ceta )


A=[cosd(ceta) , (-1*sind(ceta)*cosd(alpha)) , (sind(ceta)*sind(alpha)) , (a*cosd(ceta)) ;...........................
    sind(ceta) , (cosd(ceta)*cosd(alpha)) ,(-1*cosd(ceta)*sind(alpha)) , (a*sind(ceta)) ;............................
    0 , sind(alpha) , cosd(alpha) , d ;..................................................................................
    0,0,0,1];

== matlab function PUMA_kinematics/inverse kinematics1/RU/ Forward kinematics1 ==
  data: a input; alpha input; A output; d input; ceta input

function  A=fk_transformation_matrix(a,alpha,d,ceta )


A=[cosd(ceta) , (-1*sind(ceta)*cosd(alpha)) , (sind(ceta)*sind(alpha)) , (a*cosd(ceta)) ;...........................
    sind(ceta) , (cosd(ceta)*cosd(alpha)) ,(-1*cosd(ceta)*sind(alpha)) , (a*sind(ceta)) ;............................
    0 , sind(alpha) , cosd(alpha) , d ;..................................................................................
    0,0,0,1];

== matlab function PUMA_kinematics/inverse kinematics1/RU/ Forward kinematics2 ==
  data: a input; alpha input; A output; d input; ceta input

function  A=fk_transformation_matrix(a,alpha,d,ceta )


A=[cosd(ceta) , (-1*sind(ceta)*cosd(alpha)) , (sind(ceta)*sind(alpha)) , (a*cosd(ceta)) ;...........................
    sind(ceta) , (cosd(ceta)*cosd(alpha)) ,(-1*cosd(ceta)*sind(alpha)) , (a*sind(ceta)) ;............................
    0 , sind(alpha) , cosd(alpha) , d ;..................................................................................
    0,0,0,1];

== matlab function PUMA_kinematics/inverse kinematics1/RU/ Forward kinematics3 ==
  data: a input; alpha input; A output; d input; ceta input

function  A=fk_transformation_matrix(a,alpha,d,ceta )


A=[cosd(ceta) , (-1*sind(ceta)*cosd(alpha)) , (sind(ceta)*sind(alpha)) , (a*cosd(ceta)) ;...........................
    sind(ceta) , (cosd(ceta)*cosd(alpha)) ,(-1*cosd(ceta)*sind(alpha)) , (a*sind(ceta)) ;............................
    0 , sind(alpha) , cosd(alpha) , d ;..................................................................................
    0,0,0,1];

== matlab function PUMA_kinematics/inverse kinematics1/tool LD ==
  data: A3_0 input; R6_3 output; A6_0 input


function  R6_3 = inverse_orientation(A3_0,A6_0)


R6_0 = A6_0(1:3,1:3);
R3_0 = A3_0(1:3,1:3);


R6_3 = (R3_0')*R6_0;
end

== matlab function PUMA_kinematics/inverse kinematics1/tool LU ==
  data: A3_0 input; R6_3 output; A6_0 input


function  R6_3 = inverse_orientation(A3_0,A6_0)


R6_0 = A6_0(1:3,1:3);
R3_0 = A3_0(1:3,1:3);


R6_3 = (R3_0')*R6_0;
end

== matlab function PUMA_kinematics/inverse kinematics1/tool RD ==
  data: A3_0 input; R6_3 output; A6_0 input


function  R6_3 = inverse_orientation(A3_0,A6_0)


R6_0 = A6_0(1:3,1:3);
R3_0 = A3_0(1:3,1:3);


R6_3 = (R3_0')*R6_0;
end

== matlab function PUMA_kinematics/inverse kinematics1/tool RU ==
  data: A3_0 input; R6_3 output; A6_0 input


function  R6_3 = inverse_orientation(A3_0,A6_0)


R6_0 = A6_0(1:3,1:3);
R3_0 = A3_0(1:3,1:3);


R6_3 = (R3_0')*R6_0;
end

== matlab function PUMA_kinematics/inverse kinematics1/tool down LD ==
  data: q4 output; R6_3 input; q5 output; q6 output


function [q4,q5,q6]  = tool_down(R6_3)

C5 = R6_3(3,3);


%for S5=0
if(C5==1)
    
q5=0;
q4=0;
q6=atan2d(R6_3(2,1),R6_3(1,1));


elseif(C5==-1)
        
q5=180;
q4=0;
q6=(-1)*(atan2d((-1)*R6_3(1,2),(-1)*R6_3(1,1)));
        
 else
% for S5<1

q5 = atan2d((-1)*(sqrt(1-C5^2)),C5);
q4=atan2d((-1)*R6_3(2,3),(-1)*R6_3(1,3));
q6=atan2d((-1)*R6_3(3,2),R6_3(3,1));

end
end

== matlab function PUMA_kinematics/inverse kinematics1/tool down RD ==
  data: R6_3 input; q4 output; q5 output; q6 output


function [q4,q5,q6]  = tool_down(R6_3)

C5 = R6_3(3,3);


%for S5=0
if(C5==1)
    
q5=0;
q4=0;
q6=atan2d(R6_3(2,1),R6_3(1,1));


elseif(C5==-1)
        
q5=180;
q4=0;
q6=(-1)*(atan2d((-1)*R6_3(1,2),(-1)*R6_3(1,1)));
        
 else
% for S5<1

q5 = atan2d((-1)*(sqrt(1-C5^2)),C5);
q4=atan2d((-1)*R6_3(2,3),(-1)*R6_3(1,3));
q6=atan2d((-1)*R6_3(3,2),R6_3(3,1));

end
end

== matlab function PUMA_kinematics/inverse kinematics1/tool up LD ==
  data: q4 output; R6_3 input; q5 output; q6 output


function [q4,q5,q6]  = tool_up(R6_3)

C5 = R6_3(3,3);


%for S5=0
if(C5==1)
    
q5=0;
q4=0;
q6=atan2d(R6_3(2,1),R6_3(1,1));


elseif(C5==-1)
        
q5=180;
q4=0;
q6=(-1)*(atan2d((-1)*R6_3(1,2),(-1)*R6_3(1,1)));
        
 else
% for S5>1

q5 = atan2d((sqrt(1-C5^2)),C5);
q4=atan2d(R6_3(2,3),R6_3(1,3));
q6=atan2d(R6_3(3,2),R6_3(3,1)*(-1));

end
end

== matlab function PUMA_kinematics/inverse kinematics1/tool up RD ==
  data: R6_3 input; q4 output; q5 output; q6 output

function [q4,q5,q6]  = tool_up(R6_3)

C5 = R6_3(3,3);


%for S5=0
if(C5==1)
    
q5=0;
q4=0;
q6=atan2d(R6_3(2,1),R6_3(1,1));


elseif(C5==-1)
        
q5=180;
q4=0;
q6=(-1)*(atan2d((-1)*R6_3(1,2),(-1)*R6_3(1,1)));
        
 else
% for S5>1

q5 = atan2d((sqrt(1-C5^2)),C5);
q4=atan2d(R6_3(2,3),R6_3(1,3));
q6=atan2d(R6_3(3,2),R6_3(3,1)*(-1));

end
end

== matlab function PUMA_kinematics/inverse kinematics1/tool down LU ==
  data: R6_3 input; q4 output; q5 output; q6 output


function [q4,q5,q6]  = tool_down(R6_3)

C5 = R6_3(3,3);


%for S5=0
if(C5==1)
    
q5=0;
q4=0;
q6=atan2d(R6_3(2,1),R6_3(1,1));


elseif(C5==-1)
        
q5=180;
q4=0;
q6=(-1)*(atan2d((-1)*R6_3(1,2),(-1)*R6_3(1,1)));
        
 else
% for S5<1

q5 = atan2d((-1)*(sqrt(1-C5^2)),C5);
q4=atan2d((-1)*R6_3(2,3),(-1)*R6_3(1,3));
q6=atan2d((-1)*R6_3(3,2),R6_3(3,1));

end
end

== matlab function PUMA_kinematics/inverse kinematics1/tool down RU ==
  data: R6_3 input; q4 output; q5 output; q6 output

function [q4,q5,q6]  = tool_down(R6_3)

C5 = R6_3(3,3);


%for S5=0
if(C5==1)
    
q5=0;
q4=0;
q6=atan2d(R6_3(2,1),R6_3(1,1));


elseif(C5==-1)
        
q5=180;
q4=0;
q6=(-1)*(atan2d((-1)*R6_3(1,2),(-1)*R6_3(1,1)));
        
 else
% for S5<1

q5 = atan2d((-1)*(sqrt(1-C5^2)),C5);
q4=atan2d((-1)*R6_3(2,3),(-1)*R6_3(1,3));
q6=atan2d((-1)*R6_3(3,2),R6_3(3,1));

end
end

== matlab function PUMA_kinematics/inverse kinematics1/tool up LU ==
  data: R6_3 input; q4 output; q5 output; q6 output


function [q4,q5,q6]  = tool_up(R6_3)

C5 = R6_3(3,3);


%for S5=0
if(C5==1)
    
q5=0;
q4=0;
q6=atan2d(R6_3(2,1),R6_3(1,1));


elseif(C5==-1)
        
q5=180;
q4=0;
q6=(-1)*(atan2d((-1)*R6_3(1,2),(-1)*R6_3(1,1)));
        
 else
% for S5>1

q5 = atan2d((sqrt(1-C5^2)),C5);
q4=atan2d(R6_3(2,3),R6_3(1,3));
q6=atan2d(R6_3(3,2),R6_3(3,1)*(-1));

end
end

== matlab function PUMA_kinematics/inverse kinematics1/tool up RU ==
  data: q4 output; R6_3 input; q5 output; q6 output

function [q4,q5,q6]  = tool_up(R6_3)

C5 = R6_3(3,3);


%for S5=0
if(C5==1)
    
q5=0;
q4=0;
q6=atan2d(R6_3(2,1),R6_3(1,1));


elseif(C5==-1)
        
q5=180;
q4=0;
q6=(-1)*(atan2d((-1)*R6_3(1,2),(-1)*R6_3(1,1)));
        
 else
% for S5>1

q5 = atan2d((sqrt(1-C5^2)),C5);
q4=atan2d(R6_3(2,3),R6_3(1,3));
q6=atan2d(R6_3(3,2),R6_3(3,1)*(-1));

end
end

== matlab function PUMA_kinematics/Forward kenmatics1/ Forward kinematics1 ==
  data: a input; alpha input; A output; d input; ceta input

function  A=fk_transformation_matrix(a,alpha,d,ceta )


A=[cosd(ceta) , (-1*sind(ceta)*cosd(alpha)) , (sind(ceta)*sind(alpha)) , (a*cosd(ceta)) ;...........................
    sind(ceta) , (cosd(ceta)*cosd(alpha)) ,(-1*cosd(ceta)*sind(alpha)) , (a*sind(ceta)) ;............................
    0 , sind(alpha) , cosd(alpha) , d ;..................................................................................
    0,0,0,1];

== matlab function PUMA_kinematics/Forward kenmatics1/ Forward kinematics2 ==
  data: a input; alpha input; A output; d input; ceta input

function  A=fk_transformation_matrix(a,alpha,d,ceta )


A=[cosd(ceta) , (-1*sind(ceta)*cosd(alpha)) , (sind(ceta)*sind(alpha)) , (a*cosd(ceta)) ;...........................
    sind(ceta) , (cosd(ceta)*cosd(alpha)) ,(-1*cosd(ceta)*sind(alpha)) , (a*sind(ceta)) ;............................
    0 , sind(alpha) , cosd(alpha) , d ;..................................................................................
    0,0,0,1];

== matlab function PUMA_kinematics/Forward kenmatics1/ Forward kinematics3 ==
  data: a input; alpha input; A output; d input; ceta input

function  A=fk_transformation_matrix(a,alpha,d,ceta )


A=[cosd(ceta) , (-1*sind(ceta)*cosd(alpha)) , (sind(ceta)*sind(alpha)) , (a*cosd(ceta)) ;...........................
    sind(ceta) , (cosd(ceta)*cosd(alpha)) ,(-1*cosd(ceta)*sind(alpha)) , (a*sind(ceta)) ;............................
    0 , sind(alpha) , cosd(alpha) , d ;..................................................................................
    0,0,0,1];

== matlab function PUMA_kinematics/Forward kenmatics1/ Forward kinematics4 ==
  data: a input; alpha input; A output; d input; ceta input

function  A=fk_transformation_matrix(a,alpha,d,ceta )


A=[cosd(ceta) , (-1*sind(ceta)*cosd(alpha)) , (sind(ceta)*sind(alpha)) , (a*cosd(ceta)) ;...........................
    sind(ceta) , (cosd(ceta)*cosd(alpha)) ,(-1*cosd(ceta)*sind(alpha)) , (a*sind(ceta)) ;............................
    0 , sind(alpha) , cosd(alpha) , d ;..................................................................................
    0,0,0,1];

== matlab function PUMA_kinematics/Forward kenmatics1/ Forward kinematics5 ==
  data: a input; alpha input; A output; d input; ceta input

function  A=fk_transformation_matrix(a,alpha,d,ceta )


A=[cosd(ceta) , (-1*sind(ceta)*cosd(alpha)) , (sind(ceta)*sind(alpha)) , (a*cosd(ceta)) ;...........................
    sind(ceta) , (cosd(ceta)*cosd(alpha)) ,(-1*cosd(ceta)*sind(alpha)) , (a*sind(ceta)) ;............................
    0 , sind(alpha) , cosd(alpha) , d ;..................................................................................
    0,0,0,1];

== matlab function PUMA_kinematics/Forward kenmatics1/ Forward kinematics6 ==
  data: a input; alpha input; A output; d input; ceta input

function  A=fk_transformation_matrix(a,alpha,d,ceta )


A=[cosd(ceta) , (-1*sind(ceta)*cosd(alpha)) , (sind(ceta)*sind(alpha)) , (a*cosd(ceta)) ;...........................
    sind(ceta) , (cosd(ceta)*cosd(alpha)) ,(-1*cosd(ceta)*sind(alpha)) , (a*sind(ceta)) ;............................
    0 , sind(alpha) , cosd(alpha) , d ;..................................................................................
    0,0,0,1];

== matlab function PUMA_kinematics/inverse kinematics1/elbow down R ==
  data: Xc input; q2 output; Yc input; Zc input; a2 input; d4 input; d1 input; d2 input; q3 output



function [q2,q3]= elbow_down(Xc,Yc,Zc,a2,d4,d1,d2)


D  = ((Xc^2)+(Yc^2)-(d2^2)+(Zc-d1)^2-(a2^2)-(d4^2))/(2*a2*d4);

q3 = atan2d(sqrt(1-(D^2)),D);

q2 = 180 + atan2d((Zc-d1),sqrt((Xc^2)+(Yc^2)-(d2^2))) - atan2d(d4*sind(q3),a2+d4*cosd(q3));

end

== matlab function PUMA_kinematics/inverse kinematics1/elbow up R ==
  data: q2 output; Xc input; Yc input; Zc input; a2 input; d4 input; d1 input; d2 input; q3 output



function [q2,q3]  = elbow_up(Xc,Yc,Zc,a2,d4,d1,d2)


D  = ((Xc^2)+(Yc^2)-(d2^2)+(Zc-d1)^2-(a2^2)-(d4^2))/(2*a2*d4);

q3 = atan2d(-1*(sqrt(1-(D^2))),D);

q2 = 180+ atan2d((Zc-d1),sqrt((Xc^2)+(Yc^2)-(d2^2))) - atan2d(d4*sind(q3),a2+d4*cosd(q3));

end

== matlab function PUMA_kinematics/inverse kinematics1/left arm ==
  data: Xc input; q1 output; Yc input; d2 input

function  q1=Left_arm(Xc,Yc,d2)


w=sqrt(Xc^2+Yc^2-d2^2);

gama = atan2d(Yc,Xc);

alpha = atan2d(d2,w);

q1 = gama-alpha;

end

== matlab function PUMA_kinematics/inverse kinematics1/wrist ==
  data: A6_0 input; Xc output; d6 input; Yc output; Zc output


function  [Xc,Yc,Zc] = wrist_center(A6_0,d6)


Ox = A6_0(1,4);
Oy = A6_0(2,4);
Oz = A6_0(3,4);

r13=A6_0(1,3);
r23=A6_0(2,3);
r33=A6_0(3,3);


Xc = Ox - (d6*r13);
Yc = Oy - (d6*r23);
Zc = Oz - (d6*r33);


end

== matlab function PUMA_kinematics/inverse kinematics1/right arm ==
  data: Xc input; q1 output; Yc input; d2 input


function q1=Right_arm(Xc,Yc,d2)

w=sqrt(Xc^2+Yc^2-d2^2);

angle1 = atan2d(Yc,Xc);

angle2 = atan2d(d2,w);

q1 = angle1+angle2+180;

end
